simulink model "alu_test_6_two_charts__to_give_final"  (Simulink 7.5)
settings: Solver=FixedStepDiscrete  StartTime=0.0  StopTime=30  FixedStep=1  RelTol=1e-3
settings Model: Creator=radud  LastModifiedBy=sreesan
settings DataIOCC: SignalLogging=off
settings OptimizationCC: BlockReduction=off  ConditionallyExecuteInputs=off  InlineParams=on
settings DebuggingCC: AlgebraicLoopMsg=error  SingleTaskRateTransMsg=error
settings HardwareCC: ProdHWDeviceType=ASIC/FPGA->ASIC/FPGA

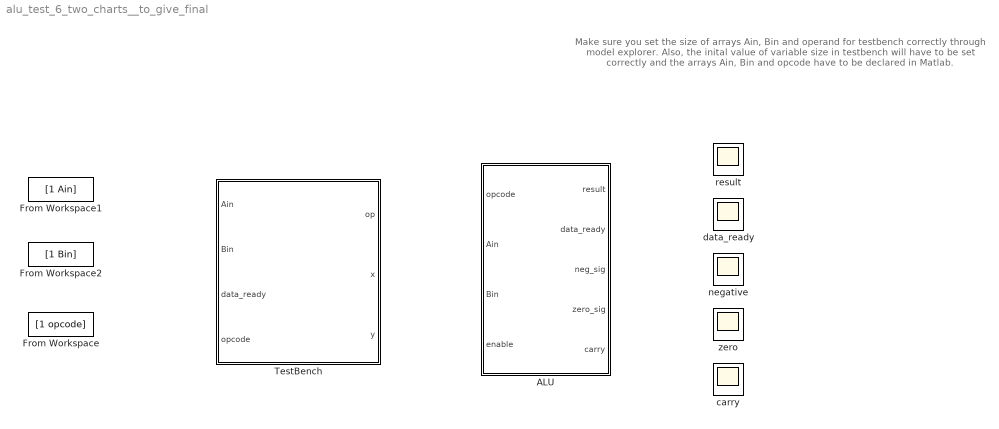
== system alu_test_6_two_charts__to_give_final ==
  note: Make sure you set the size of arrays Ain, Bin and operand
      | for testbench correctly through model explorer.
      | Also, the inital value of variable size in
      | testbench will have to be set correctly and
      | the arrays Ain, Bin and opcode have to be declared in Matlab.
  ALU : Stateflow chart  TreatAsAtomicUnit=on
  From Workspace : FromWorkspace  VariableName=[1 opcode]  SampleTime=0  Interpolate=off  OutputAfterFinalValue=Holding final value
  From Workspace1 : FromWorkspace  VariableName=[1 Ain]  SampleTime=1  OutputAfterFinalValue=Holding final value
  From Workspace2 : FromWorkspace  VariableName=[1 Bin]  SampleTime=1  OutputAfterFinalValue=Holding final value
  TestBench : Stateflow chart  TreatAsAtomicUnit=on
  carry : Scope
      settings: YMin=0  YMax=80
  data_ready : Scope
      settings: YMin=0  YMax=80  SaveName=ScopeData4
  negative : Scope
      settings: YMin=0  YMax=80  SaveName=ScopeData2
  result : Scope
      settings: YMin=0  YMax=80
  zero : Scope
      settings: YMin=0  YMax=80  SaveName=ScopeData3

== stateflow chart ALU ==
  settings: executeAtInitialization=1
  state ALU [parallel]
    settings: executionOrder=1
  data: opcode input uint8; result output int16; Ain input int8; Bin input int8; data_ready output boolean; enable input boolean; neg_sig output boolean; zero_sig output boolean; carry output boolean

== stateflow chart TestBench ==
  settings: executeAtInitialization=1
  state testbench [parallel]
    settings: executionOrder=1
    state idle
      en:
      op=op_temp;
      x=Ain[i];
      y=Bin[j];
      i=i+1;
      j=j+1;
    state data
      en:
      op_temp=opcode[i];
    state start
      en:
    state idle1
      en:
      op=op_temp;
      x=Ain[i];
      i=i+1;
    idle -> data : [i<size && data_ready==1]
    data -> (junction 20)
    (default) -> start
    start -> data
    (junction 20) -> idle [order 1] : [op_temp<5]
    (junction 20) -> idle1 [order 2] : [op_temp>=5 && op_temp<7]
    idle1 -> data : [i<size && data_ready==1]
  data: Ain input int8 size=7 =[1 4 6 8 3]; Bin input int8 size=5 =[1 2 3 4 5]; data_ready input double; i local double; op output uint8 =-1; opcode input uint8 size=7 =[0 1 2 3 4]; x output int8; y output int8; j local double; size local double =7; op_temp local uint8
